simulink model "simu"  (R2018b)
settings: Solver=VariableStepAuto  StartTime=0.0  StopTime=10  RelTol=1e-3
values from neighbouring files (symbols this model uses):
  Ad = SYSD.A    [Main.m]
  Ao = Sys_Obs.A    [Main.m]
  Bd = SYSD.B    [Main.m]
  Bo = Sys_Obs.B    [Main.m]
  Cd = SYSD.C    [Main.m]
  Fd = dlqr(Ad,Bd,Qc ,1)    [Main.m]
  fe = 1000    [Main.m]
  G = inv(Cd*inv(eye(2)-Ad+Bd*Fd)*Bd)    [Main.m]
  Kp = 5    [Main.m]
  SYS = ss(A,B,C,D)    [Main.m]
settings Model: Creator=piffercg  LastModifiedBy=piffercg

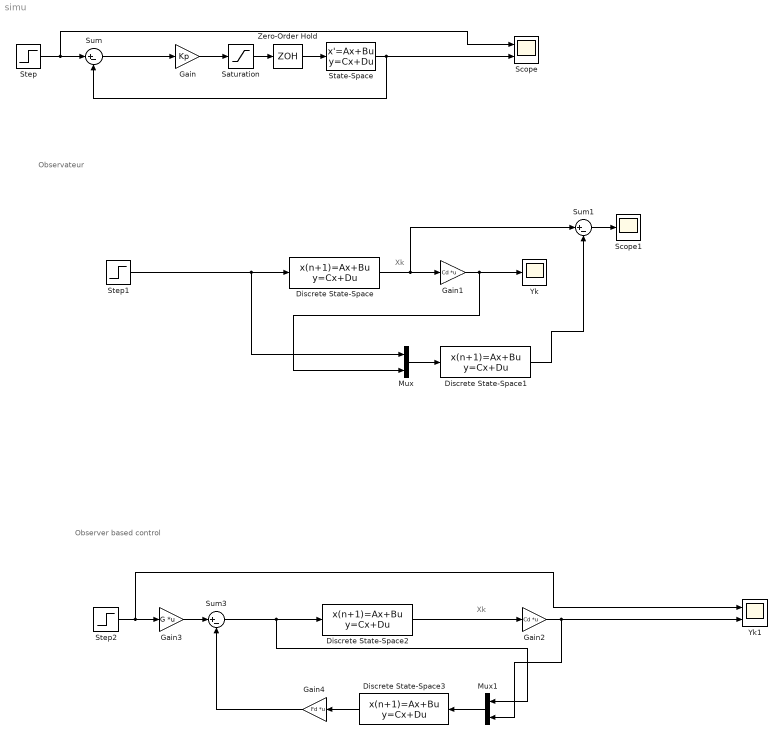
== system simu ==
  note: Observer based control
  note: Xk
  note: Observateur
  note: Xk
  Discrete State-Space : DiscreteStateSpace  A=Ad  B=Bd  C=eye(2)  D=zeros(2,1)  SampleTime=1/fe
  Discrete State-Space1 : DiscreteStateSpace  A=Ao  B=Bo  C=eye(2)  D=zeros(2,2)  InitialCondition=0.001  SampleTime=1/fe
  Discrete State-Space2 : DiscreteStateSpace  A=Ad  B=Bd  C=eye(2)  D=zeros(2,1)  SampleTime=1/fe
  Discrete State-Space3 : DiscreteStateSpace  A=Ao  B=Bo  C=eye(2)  D=zeros(2,2)  InitialCondition=0.001  SampleTime=1/fe
  Gain : Gain  Gain=Kp
  Gain1 : Gain  Gain=Cd  Multiplication=Matrix(K*u)
  Gain2 : Gain  Gain=Cd  Multiplication=Matrix(K*u)
  Gain3 : Gain  Gain=G  Multiplication=Matrix(K*u)
  Gain4 : Gain  Gain=Fd  Multiplication=Matrix(K*u)
  Mux : Mux  Inputs=2
  Mux1 : Mux  Inputs=2
  Saturation : Saturate  UpperLimit=10  LowerLimit=-10
  Scope : Scope  NumInputPorts=2
  Scope1 : Scope
  State-Space : StateSpace  A=SYS.A  B=SYS.B  C=SYS.C  D=SYS.D  InitialCondition=0
  Step : Step  SampleTime=0
  Step1 : Step  SampleTime=0
  Step2 : Step  SampleTime=0
  Sum : Sum  Inputs=|+-
  Sum1 : Sum  Inputs=|+-
  Sum3 : Sum  Inputs=|+-
  Yk : Scope
  Yk1 : Scope  NumInputPorts=2
  Zero-Order Hold : ZeroOrderHold  SampleTime=1/fe
  wires:
  Step/1 -> Scope/1, Sum/1
  Sum/1 -> Gain/1
  State-Space/1 -> Sum/2, Scope/2
  Gain/1 -> Saturation/1
  Saturation/1 -> Zero-Order Hold/1
  Zero-Order Hold/1 -> State-Space/1
  Discrete State-Space/1 -> Sum1/1, Gain1/1
  Gain1/1 -> Mux/2, Yk/1
  Mux/1 -> Discrete State-Space1/1
  Step1/1 -> Mux/1, Discrete State-Space/1
  Discrete State-Space1/1 -> Sum1/2
  Sum1/1 -> Scope1/1
  Gain2/1 -> Yk1/2, Mux1/2
  Discrete State-Space2/1 -> Gain2/1
  Mux1/1 -> Discrete State-Space3/1
  Step2/1 -> Yk1/1, Gain3/1
  Gain3/1 -> Sum3/1
  Discrete State-Space3/1 -> Gain4/1
  Gain4/1 -> Sum3/2
  Sum3/1 -> Mux1/1, Discrete State-Space2/1
